simulink library "ComputeNormalSurface"  (R2014b)
settings: Solver=ode45  StartTime=0.0  StopTime=10.0  RelTol=1e-3
settings Model: Creator=Hp  LastModifiedBy=Hp

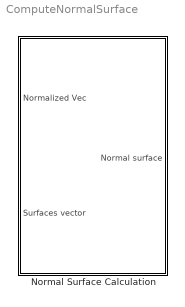
== system ComputeNormalSurface ==
  Normal Surface Calculation : Subsystem

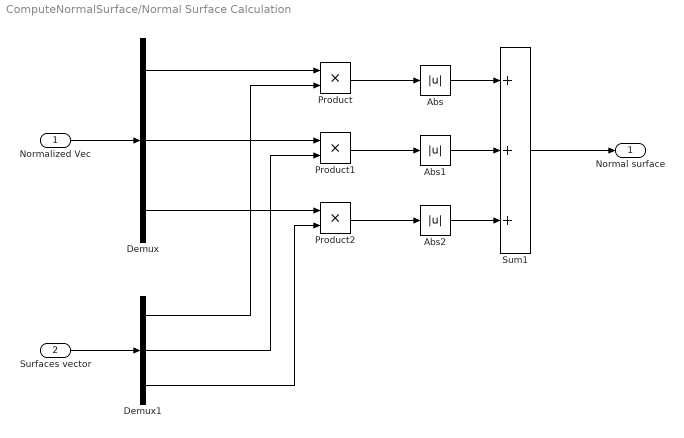
== system ComputeNormalSurface/Normal Surface Calculation ==
  "Normalized Vec " : Inport
  Surfaces vector : Inport  Port=2
  Abs : Abs
  Abs1 : Abs
  Abs2 : Abs
  Demux : Demux  Outputs=3
  Demux1 : Demux  Outputs=3
  Product : Product
  Product1 : Product
  Product2 : Product
  Sum1 : Sum  Inputs=+++
  Normal surface : Outport
  wires:
  Abs/1 -> Sum1/1
  Demux/3 -> Product2/1
  Demux/2 -> Product1/1
  Demux1/1 -> Product/2
  Sum1/1 -> Normal surface/1
  "Normalized Vec "/1 -> Demux/1
  Abs1/1 -> Sum1/2
  Product/1 -> Abs/1
  Product2/1 -> Abs2/1
  Surfaces vector/1 -> Demux1/1
  Demux1/2 -> Product1/2
  Demux1/3 -> Product2/2
  Product1/1 -> Abs1/1
  Abs2/1 -> Sum1/3
  Demux/1 -> Product/1
